simulink model "check_time"  (R2013a)
settings: Solver=ode3  StartTime=0.0  StopTime=T  FixedStep=t_samples  RelTol=1e-3
values from neighbouring files (symbols this model uses):
  t_samples = 0.1    [wide_trajectory.mat]
settings Model: Creator=HP  LastModifiedBy=HP

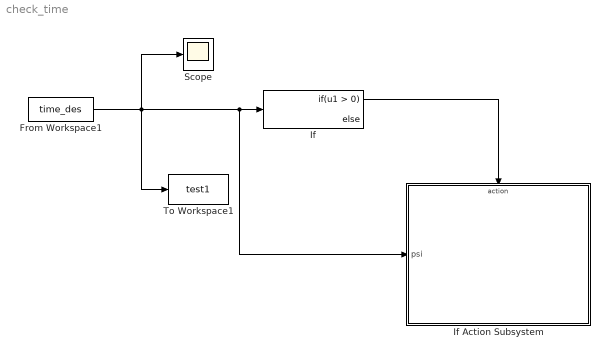
== system check_time ==
  From Workspace1 : FromWorkspace  VariableName=time_des  SampleTime=t_samples
  If : If  SampleTime=t_samples
  If Action Subsystem : Subsystem  TreatAsAtomicUnit=on
  Scope : Scope
  To Workspace1 : ToWorkspace  VariableName=test1  SampleTime=t_samples
  wires:
  If/1 -> If Action Subsystem/Action
  From Workspace1/1 -> To Workspace1/1, Scope/1, If Action Subsystem/1(psi), If/1

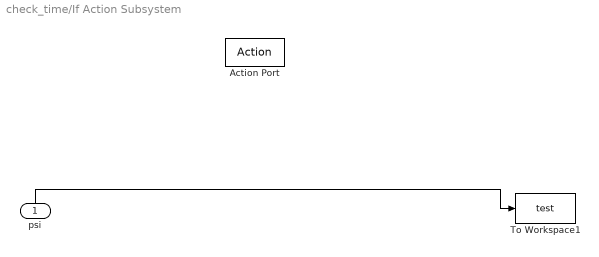
== system check_time/If Action Subsystem ==
  psi : Inport
  Action Port : ActionPort  ActionType=then
  To Workspace1 : ToWorkspace  VariableName=test  SampleTime=t_samples  SaveFormat=Structure With Time
  wires:
  psi/1 -> To Workspace1/1
